simulink model "COSTEP_Auto"  (R2024b)
settings: Solver=FixedStepAuto  StartTime=0.0  StopTime=25  FixedStep=1/3600  RelTol=1e-3
model workspace (MAT data in the model file):
  AD : Simulink.Parameter (value not decoded)
  AG : Simulink.Parameter (value not decoded)
  AH : Simulink.Parameter (value not decoded)
  AV : Simulink.Parameter (value not decoded)
  AVP : Simulink.Parameter (value not decoded)
  BCHL : Simulink.Parameter (value not decoded)
  BCHV : Simulink.Parameter (value not decoded)
  BD : Simulink.Parameter (value not decoded)
  BG : Simulink.Parameter (value not decoded)
  BH : Simulink.Parameter (value not decoded)
  BVP : Simulink.Parameter (value not decoded)
  CD : Simulink.Parameter (value not decoded)
  CG : Simulink.Parameter (value not decoded)
  CH : Simulink.Parameter (value not decoded)
  CVP : Simulink.Parameter (value not decoded)
  ISV : Simulink.Parameter (value not decoded)
  XMW : Simulink.Parameter (value not decoded)
  XNS : Simulink.Parameter (value not decoded)
  XNS2 : Simulink.Parameter (value not decoded)
  XNS3 : Simulink.Parameter (value not decoded)
  XNSE : Simulink.Parameter (value not decoded)
values from neighbouring files (symbols this model uses):
  DD = SimData{4,1}{1,2}    [Auto_run_COSTEP.m]    (also in Run_COSTEP.m)
  G = SimData{2,1}(j,2)    [Auto_run_COSTEP.m]    (also in G.mat = [4243534565 7854912354 3456432354 1731738903 4346024432 5784; Run_COSTEP.m)
  IDV = SimData{3,1}(1:20,j)    [Auto_run_COSTEP.m]    (also in IDV.mat = [0 0 0 0 0 0 0 0 0 0 0 0 ... (812 elements, 28x29)]; Run_COSTEP.m = SimData{3,1}(1:28,j))
symbols that are objects in the model workspace (value not decoded): AD, AG, AH, AV, AVP, BD, BG, BH, BVP, CD, CG, CH, CVP, XMW, XNS, XNS2, XNS3, XNSE
undefined symbols (not defined in the file or in its folder): magnitude, msgbox, SETPT, XMEAS, XMV
libraries: mylib x304, dspindex x31
(part 11 of 13)

== system COSTEP_Auto/Control Mode/Ricker/Subsystem8/Control Loop 11/PI Control Measurement Velocity form/Subsystem ==
  Setpoint : Inport
  Measurement : Inport  Port=2
  Controller Gain : Gain  Gain=Kc  SaturateOnIntegerOverflow=on  OutDataTypeStr=Inherit: Same as input  ParamDataTypeStr=Inherit: Same as input
  Error : ZeroOrderHold  SampleTime=Ts
  Error old : UnitDelay  SampleTime=Ts
  Gain1 : Gain  Gain=Ts/Ti  SaturateOnIntegerOverflow=on  OutDataTypeStr=Inherit: Same as input  ParamDataTypeStr=Inherit: Same as input
  Sum : Sum  Inputs=|+-  SaturateOnIntegerOverflow=on
  Sum1 : Sum  Inputs=++-  SaturateOnIntegerOverflow=on
  Delta Output : Outport
  wires:
  Measurement/1 -> Sum/2
  Controller Gain/1 -> Delta Output/1
  Gain1/1 -> Sum1/2
  Setpoint/1 -> Sum/1
  Error old/1 -> Sum1/3
  Sum1/1 -> Controller Gain/1
  Error/1 -> Sum1/1, Error old/1, Gain1/1
  Sum/1 -> Error/1

== system COSTEP_Auto/Random number generator/Stream Measurements SMEAS Gas analysis/If Action Subsystem3/Subsystem/Stream 1/Subsystem ==
  G : Inport
  TESUB6 XMNSEA : Subsystem
  TESUB6 XMNSEB : Subsystem
  TESUB6 XMNSEC : Subsystem
  TESUB6 XMNSED : Subsystem
  TESUB6 XMNSEE : Subsystem
  TESUB6 XMNSEF : Subsystem
  TESUB6 XMNSEG : Subsystem
  TESUB6 XMNSEH : Subsystem
  XMNSEA : Outport  VectorParamsAs1DForOutWhenUnconnected=off
  XMNSEB : Outport  Port=2  VectorParamsAs1DForOutWhenUnconnected=off
  XMNSEC : Outport  Port=3  VectorParamsAs1DForOutWhenUnconnected=off
  XMNSED : Outport  Port=4  VectorParamsAs1DForOutWhenUnconnected=off
  XMNSEE : Outport  Port=5  VectorParamsAs1DForOutWhenUnconnected=off
  XMNSEF : Outport  Port=6  VectorParamsAs1DForOutWhenUnconnected=off
  XMNSEG : Outport  Port=7  VectorParamsAs1DForOutWhenUnconnected=off
  XMNSEH : Outport  Port=8  VectorParamsAs1DForOutWhenUnconnected=off
  G_NEW : Outport  Port=9  VectorParamsAs1DForOutWhenUnconnected=off
  wires:
  TESUB6 XMNSEB/2(G_NEW) -> TESUB6 XMNSEC/1(G)
  G/1 -> TESUB6 XMNSEA/1(G)
  TESUB6 XMNSEA/2(G_NEW) -> TESUB6 XMNSEB/1(G)
  TESUB6 XMNSEC/2(G_NEW) -> TESUB6 XMNSED/1(G)
  TESUB6 XMNSED/1(XMNSED) -> XMNSED/1  "XMNSED"
  TESUB6 XMNSEE/1(XMNSEE) -> XMNSEE/1  "XMNSEE"
  TESUB6 XMNSED/2(G_NEW) -> TESUB6 XMNSEE/1(G)
  TESUB6 XMNSEC/1(XMNSEC) -> XMNSEC/1  "XMNSEC"
  TESUB6 XMNSEA/1(XMNSEA) -> XMNSEA/1  "XMNSEA"
  TESUB6 XMNSEB/1(XMNSEB) -> XMNSEB/1  "XMNSEB"
  TESUB6 XMNSEE/2(G_NEW) -> TESUB6 XMNSEF/1(G)
  TESUB6 XMNSEF/2(G_NEW) -> TESUB6 XMNSEG/1(G)
  TESUB6 XMNSEG/2(G_NEW) -> TESUB6 XMNSEH/1(G)
  TESUB6 XMNSEH/2(G_NEW) -> G_NEW/1
  TESUB6 XMNSEF/1(XMNSEF) -> XMNSEF/1  "XMNSEF"
  TESUB6 XMNSEG/1(XMNSEG) -> XMNSEG/1  "XMNSEG"
  TESUB6 XMNSEH/1(XMNSEH) -> XMNSEH/1  "XMNSEH"

== system COSTEP_Auto/Random number generator/Stream Measurements SMEAS Gas analysis/If Action Subsystem3/Subsystem/Stream 13/Subsystem ==
  G : Inport
  TESUB6 XMNSEA : Subsystem
  TESUB6 XMNSEB : Subsystem
  TESUB6 XMNSEC : Subsystem
  TESUB6 XMNSED : Subsystem
  TESUB6 XMNSEE : Subsystem
  TESUB6 XMNSEF : Subsystem
  TESUB6 XMNSEG : Subsystem
  TESUB6 XMNSEH : Subsystem
  XMNSEA : Outport  VectorParamsAs1DForOutWhenUnconnected=off
  XMNSEB : Outport  Port=2  VectorParamsAs1DForOutWhenUnconnected=off
  XMNSEC : Outport  Port=3  VectorParamsAs1DForOutWhenUnconnected=off
  XMNSED : Outport  Port=4  VectorParamsAs1DForOutWhenUnconnected=off
  XMNSEE : Outport  Port=5  VectorParamsAs1DForOutWhenUnconnected=off
  XMNSEF : Outport  Port=6  VectorParamsAs1DForOutWhenUnconnected=off
  XMNSEG : Outport  Port=7  VectorParamsAs1DForOutWhenUnconnected=off
  XMNSEH : Outport  Port=8  VectorParamsAs1DForOutWhenUnconnected=off
  G_NEW : Outport  Port=9  VectorParamsAs1DForOutWhenUnconnected=off
  wires:
  TESUB6 XMNSEB/2(G_NEW) -> TESUB6 XMNSEC/1(G)
  G/1 -> TESUB6 XMNSEA/1(G)
  TESUB6 XMNSEA/2(G_NEW) -> TESUB6 XMNSEB/1(G)
  TESUB6 XMNSEC/2(G_NEW) -> TESUB6 XMNSED/1(G)
  TESUB6 XMNSED/1(XMNSED) -> XMNSED/1  "XMNSED"
  TESUB6 XMNSEE/1(XMNSEE) -> XMNSEE/1  "XMNSEE"
  TESUB6 XMNSED/2(G_NEW) -> TESUB6 XMNSEE/1(G)
  TESUB6 XMNSEC/1(XMNSEC) -> XMNSEC/1  "XMNSEC"
  TESUB6 XMNSEA/1(XMNSEA) -> XMNSEA/1  "XMNSEA"
  TESUB6 XMNSEB/1(XMNSEB) -> XMNSEB/1  "XMNSEB"
  TESUB6 XMNSEE/2(G_NEW) -> TESUB6 XMNSEF/1(G)
  TESUB6 XMNSEF/2(G_NEW) -> TESUB6 XMNSEG/1(G)
  TESUB6 XMNSEG/2(G_NEW) -> TESUB6 XMNSEH/1(G)
  TESUB6 XMNSEH/2(G_NEW) -> G_NEW/1
  TESUB6 XMNSEF/1(XMNSEF) -> XMNSEF/1  "XMNSEF"
  TESUB6 XMNSEG/1(XMNSEG) -> XMNSEG/1  "XMNSEG"
  TESUB6 XMNSEH/1(XMNSEH) -> XMNSEH/1  "XMNSEH"

== system COSTEP_Auto/Random number generator/Stream Measurements SMEAS Gas analysis/If Action Subsystem3/Subsystem/Stream 2/Subsystem ==
  G : Inport
  TESUB6 XMNSEA : Subsystem
  TESUB6 XMNSEB : Subsystem
  TESUB6 XMNSEC : Subsystem
  TESUB6 XMNSED : Subsystem
  TESUB6 XMNSEE : Subsystem
  TESUB6 XMNSEF : Subsystem
  TESUB6 XMNSEG : Subsystem
  TESUB6 XMNSEH : Subsystem
  XMNSEA : Outport  VectorParamsAs1DForOutWhenUnconnected=off
  XMNSEB : Outport  Port=2  VectorParamsAs1DForOutWhenUnconnected=off
  XMNSEC : Outport  Port=3  VectorParamsAs1DForOutWhenUnconnected=off
  XMNSED : Outport  Port=4  VectorParamsAs1DForOutWhenUnconnected=off
  XMNSEE : Outport  Port=5  VectorParamsAs1DForOutWhenUnconnected=off
  XMNSEF : Outport  Port=6  VectorParamsAs1DForOutWhenUnconnected=off
  XMNSEG : Outport  Port=7  VectorParamsAs1DForOutWhenUnconnected=off
  XMNSEH : Outport  Port=8  VectorParamsAs1DForOutWhenUnconnected=off
  G_NEW : Outport  Port=9  VectorParamsAs1DForOutWhenUnconnected=off
  wires:
  TESUB6 XMNSEB/2(G_NEW) -> TESUB6 XMNSEC/1(G)
  G/1 -> TESUB6 XMNSEA/1(G)
  TESUB6 XMNSEA/2(G_NEW) -> TESUB6 XMNSEB/1(G)
  TESUB6 XMNSEC/2(G_NEW) -> TESUB6 XMNSED/1(G)
  TESUB6 XMNSED/1(XMNSED) -> XMNSED/1  "XMNSED"
  TESUB6 XMNSEE/1(XMNSEE) -> XMNSEE/1  "XMNSEE"
  TESUB6 XMNSED/2(G_NEW) -> TESUB6 XMNSEE/1(G)
  TESUB6 XMNSEC/1(XMNSEC) -> XMNSEC/1  "XMNSEC"
  TESUB6 XMNSEA/1(XMNSEA) -> XMNSEA/1  "XMNSEA"
  TESUB6 XMNSEB/1(XMNSEB) -> XMNSEB/1  "XMNSEB"
  TESUB6 XMNSEE/2(G_NEW) -> TESUB6 XMNSEF/1(G)
  TESUB6 XMNSEF/2(G_NEW) -> TESUB6 XMNSEG/1(G)
  TESUB6 XMNSEG/2(G_NEW) -> TESUB6 XMNSEH/1(G)
  TESUB6 XMNSEH/2(G_NEW) -> G_NEW/1
  TESUB6 XMNSEF/1(XMNSEF) -> XMNSEF/1  "XMNSEF"
  TESUB6 XMNSEG/1(XMNSEG) -> XMNSEG/1  "XMNSEG"
  TESUB6 XMNSEH/1(XMNSEH) -> XMNSEH/1  "XMNSEH"

== system COSTEP_Auto/Random number generator/Stream Measurements SMEAS Gas analysis/If Action Subsystem3/Subsystem/Stream 3/Subsystem ==
  G : Inport
  TESUB6 XMNSEA : Subsystem
  TESUB6 XMNSEB : Subsystem
  TESUB6 XMNSEC : Subsystem
  TESUB6 XMNSED : Subsystem
  TESUB6 XMNSEE : Subsystem
  TESUB6 XMNSEF : Subsystem
  TESUB6 XMNSEG : Subsystem
  TESUB6 XMNSEH : Subsystem
  XMNSEA : Outport  VectorParamsAs1DForOutWhenUnconnected=off
  XMNSEB : Outport  Port=2  VectorParamsAs1DForOutWhenUnconnected=off
  XMNSEC : Outport  Port=3  VectorParamsAs1DForOutWhenUnconnected=off
  XMNSED : Outport  Port=4  VectorParamsAs1DForOutWhenUnconnected=off
  XMNSEE : Outport  Port=5  VectorParamsAs1DForOutWhenUnconnected=off
  XMNSEF : Outport  Port=6  VectorParamsAs1DForOutWhenUnconnected=off
  XMNSEG : Outport  Port=7  VectorParamsAs1DForOutWhenUnconnected=off
  XMNSEH : Outport  Port=8  VectorParamsAs1DForOutWhenUnconnected=off
  G_NEW : Outport  Port=9  VectorParamsAs1DForOutWhenUnconnected=off
  wires:
  TESUB6 XMNSEB/2(G_NEW) -> TESUB6 XMNSEC/1(G)
  G/1 -> TESUB6 XMNSEA/1(G)
  TESUB6 XMNSEA/2(G_NEW) -> TESUB6 XMNSEB/1(G)
  TESUB6 XMNSEC/2(G_NEW) -> TESUB6 XMNSED/1(G)
  TESUB6 XMNSED/1(XMNSED) -> XMNSED/1  "XMNSED"
  TESUB6 XMNSEE/1(XMNSEE) -> XMNSEE/1  "XMNSEE"
  TESUB6 XMNSED/2(G_NEW) -> TESUB6 XMNSEE/1(G)
  TESUB6 XMNSEC/1(XMNSEC) -> XMNSEC/1  "XMNSEC"
  TESUB6 XMNSEA/1(XMNSEA) -> XMNSEA/1  "XMNSEA"
  TESUB6 XMNSEB/1(XMNSEB) -> XMNSEB/1  "XMNSEB"
  TESUB6 XMNSEE/2(G_NEW) -> TESUB6 XMNSEF/1(G)
  TESUB6 XMNSEF/2(G_NEW) -> TESUB6 XMNSEG/1(G)
  TESUB6 XMNSEG/2(G_NEW) -> TESUB6 XMNSEH/1(G)
  TESUB6 XMNSEH/2(G_NEW) -> G_NEW/1
  TESUB6 XMNSEF/1(XMNSEF) -> XMNSEF/1  "XMNSEF"
  TESUB6 XMNSEG/1(XMNSEG) -> XMNSEG/1  "XMNSEG"
  TESUB6 XMNSEH/1(XMNSEH) -> XMNSEH/1  "XMNSEH"

== system COSTEP_Auto/Random number generator/Stream Measurements SMEAS Gas analysis/If Action Subsystem3/Subsystem/Stream 4/Subsystem ==
  G : Inport
  TESUB6 XMNSEA : Subsystem
  TESUB6 XMNSEB : Subsystem
  TESUB6 XMNSEC : Subsystem
  TESUB6 XMNSED : Subsystem
  TESUB6 XMNSEE : Subsystem
  TESUB6 XMNSEF : Subsystem
  TESUB6 XMNSEG : Subsystem
  TESUB6 XMNSEH : Subsystem
  XMNSEA : Outport  VectorParamsAs1DForOutWhenUnconnected=off
  XMNSEB : Outport  Port=2  VectorParamsAs1DForOutWhenUnconnected=off
  XMNSEC : Outport  Port=3  VectorParamsAs1DForOutWhenUnconnected=off
  XMNSED : Outport  Port=4  VectorParamsAs1DForOutWhenUnconnected=off
  XMNSEE : Outport  Port=5  VectorParamsAs1DForOutWhenUnconnected=off
  XMNSEF : Outport  Port=6  VectorParamsAs1DForOutWhenUnconnected=off
  XMNSEG : Outport  Port=7  VectorParamsAs1DForOutWhenUnconnected=off
  XMNSEH : Outport  Port=8  VectorParamsAs1DForOutWhenUnconnected=off
  G_NEW : Outport  Port=9  VectorParamsAs1DForOutWhenUnconnected=off
  wires:
  TESUB6 XMNSEB/2(G_NEW) -> TESUB6 XMNSEC/1(G)
  G/1 -> TESUB6 XMNSEA/1(G)
  TESUB6 XMNSEA/2(G_NEW) -> TESUB6 XMNSEB/1(G)
  TESUB6 XMNSEC/2(G_NEW) -> TESUB6 XMNSED/1(G)
  TESUB6 XMNSED/1(XMNSED) -> XMNSED/1  "XMNSED"
  TESUB6 XMNSEE/1(XMNSEE) -> XMNSEE/1  "XMNSEE"
  TESUB6 XMNSED/2(G_NEW) -> TESUB6 XMNSEE/1(G)
  TESUB6 XMNSEC/1(XMNSEC) -> XMNSEC/1  "XMNSEC"
  TESUB6 XMNSEA/1(XMNSEA) -> XMNSEA/1  "XMNSEA"
  TESUB6 XMNSEB/1(XMNSEB) -> XMNSEB/1  "XMNSEB"
  TESUB6 XMNSEE/2(G_NEW) -> TESUB6 XMNSEF/1(G)
  TESUB6 XMNSEF/2(G_NEW) -> TESUB6 XMNSEG/1(G)
  TESUB6 XMNSEG/2(G_NEW) -> TESUB6 XMNSEH/1(G)
  TESUB6 XMNSEH/2(G_NEW) -> G_NEW/1
  TESUB6 XMNSEF/1(XMNSEF) -> XMNSEF/1  "XMNSEF"
  TESUB6 XMNSEG/1(XMNSEG) -> XMNSEG/1  "XMNSEG"
  TESUB6 XMNSEH/1(XMNSEH) -> XMNSEH/1  "XMNSEH"

== system COSTEP_Auto/Random number generator/Stream Measurements SMEAS Gas analysis/If Action Subsystem3/Subsystem/Stream 5/Subsystem ==
  G : Inport
  TESUB6 XMNSEA : Subsystem
  TESUB6 XMNSEB : Subsystem
  TESUB6 XMNSEC : Subsystem
  TESUB6 XMNSED : Subsystem
  TESUB6 XMNSEE : Subsystem
  TESUB6 XMNSEF : Subsystem
  TESUB6 XMNSEG : Subsystem
  TESUB6 XMNSEH : Subsystem
  XMNSEA : Outport  VectorParamsAs1DForOutWhenUnconnected=off
  XMNSEB : Outport  Port=2  VectorParamsAs1DForOutWhenUnconnected=off
  XMNSEC : Outport  Port=3  VectorParamsAs1DForOutWhenUnconnected=off
  XMNSED : Outport  Port=4  VectorParamsAs1DForOutWhenUnconnected=off
  XMNSEE : Outport  Port=5  VectorParamsAs1DForOutWhenUnconnected=off
  XMNSEF : Outport  Port=6  VectorParamsAs1DForOutWhenUnconnected=off
  XMNSEG : Outport  Port=7  VectorParamsAs1DForOutWhenUnconnected=off
  XMNSEH : Outport  Port=8  VectorParamsAs1DForOutWhenUnconnected=off
  G_NEW : Outport  Port=9  VectorParamsAs1DForOutWhenUnconnected=off
  wires:
  TESUB6 XMNSEB/2(G_NEW) -> TESUB6 XMNSEC/1(G)
  G/1 -> TESUB6 XMNSEA/1(G)
  TESUB6 XMNSEA/2(G_NEW) -> TESUB6 XMNSEB/1(G)
  TESUB6 XMNSEC/2(G_NEW) -> TESUB6 XMNSED/1(G)
  TESUB6 XMNSED/1(XMNSED) -> XMNSED/1  "XMNSED"
  TESUB6 XMNSEE/1(XMNSEE) -> XMNSEE/1  "XMNSEE"
  TESUB6 XMNSED/2(G_NEW) -> TESUB6 XMNSEE/1(G)
  TESUB6 XMNSEC/1(XMNSEC) -> XMNSEC/1  "XMNSEC"
  TESUB6 XMNSEA/1(XMNSEA) -> XMNSEA/1  "XMNSEA"
  TESUB6 XMNSEB/1(XMNSEB) -> XMNSEB/1  "XMNSEB"
  TESUB6 XMNSEE/2(G_NEW) -> TESUB6 XMNSEF/1(G)
  TESUB6 XMNSEF/2(G_NEW) -> TESUB6 XMNSEG/1(G)
  TESUB6 XMNSEG/2(G_NEW) -> TESUB6 XMNSEH/1(G)
  TESUB6 XMNSEH/2(G_NEW) -> G_NEW/1
  TESUB6 XMNSEF/1(XMNSEF) -> XMNSEF/1  "XMNSEF"
  TESUB6 XMNSEG/1(XMNSEG) -> XMNSEG/1  "XMNSEG"
  TESUB6 XMNSEH/1(XMNSEH) -> XMNSEH/1  "XMNSEH"

== system COSTEP_Auto/Random number generator/Stream Measurements SMEAS Gas analysis/If Action Subsystem3/Subsystem/Stream 6/Subsystem ==
  G : Inport
  TESUB6 XMNSEA : Subsystem
  TESUB6 XMNSEB : Subsystem
  TESUB6 XMNSEC : Subsystem
  TESUB6 XMNSED : Subsystem
  TESUB6 XMNSEE : Subsystem
  TESUB6 XMNSEF : Subsystem
  TESUB6 XMNSEG : Subsystem
  TESUB6 XMNSEH : Subsystem
  XMNSEA : Outport  VectorParamsAs1DForOutWhenUnconnected=off
  XMNSEB : Outport  Port=2  VectorParamsAs1DForOutWhenUnconnected=off
  XMNSEC : Outport  Port=3  VectorParamsAs1DForOutWhenUnconnected=off
  XMNSED : Outport  Port=4  VectorParamsAs1DForOutWhenUnconnected=off
  XMNSEE : Outport  Port=5  VectorParamsAs1DForOutWhenUnconnected=off
  XMNSEF : Outport  Port=6  VectorParamsAs1DForOutWhenUnconnected=off
  XMNSEG : Outport  Port=7  VectorParamsAs1DForOutWhenUnconnected=off
  XMNSEH : Outport  Port=8  VectorParamsAs1DForOutWhenUnconnected=off
  G_NEW : Outport  Port=9  VectorParamsAs1DForOutWhenUnconnected=off
  wires:
  TESUB6 XMNSEB/2(G_NEW) -> TESUB6 XMNSEC/1(G)
  G/1 -> TESUB6 XMNSEA/1(G)
  TESUB6 XMNSEA/2(G_NEW) -> TESUB6 XMNSEB/1(G)
  TESUB6 XMNSEC/2(G_NEW) -> TESUB6 XMNSED/1(G)
  TESUB6 XMNSED/1(XMNSED) -> XMNSED/1  "XMNSED"
  TESUB6 XMNSEE/1(XMNSEE) -> XMNSEE/1  "XMNSEE"
  TESUB6 XMNSED/2(G_NEW) -> TESUB6 XMNSEE/1(G)
  TESUB6 XMNSEC/1(XMNSEC) -> XMNSEC/1  "XMNSEC"
  TESUB6 XMNSEA/1(XMNSEA) -> XMNSEA/1  "XMNSEA"
  TESUB6 XMNSEB/1(XMNSEB) -> XMNSEB/1  "XMNSEB"
  TESUB6 XMNSEE/2(G_NEW) -> TESUB6 XMNSEF/1(G)
  TESUB6 XMNSEF/2(G_NEW) -> TESUB6 XMNSEG/1(G)
  TESUB6 XMNSEG/2(G_NEW) -> TESUB6 XMNSEH/1(G)
  TESUB6 XMNSEH/2(G_NEW) -> G_NEW/1
  TESUB6 XMNSEF/1(XMNSEF) -> XMNSEF/1  "XMNSEF"
  TESUB6 XMNSEG/1(XMNSEG) -> XMNSEG/1  "XMNSEG"
  TESUB6 XMNSEH/1(XMNSEH) -> XMNSEH/1  "XMNSEH"

== system COSTEP_Auto/Random number generator/Stream Measurements SMEAS Gas analysis/If Action Subsystem3/Subsystem/Stream 8/Subsystem ==
  G : Inport
  TESUB6 XMNSEA : Subsystem
  TESUB6 XMNSEB : Subsystem
  TESUB6 XMNSEC : Subsystem
  TESUB6 XMNSED : Subsystem
  TESUB6 XMNSEE : Subsystem
  TESUB6 XMNSEF : Subsystem
  TESUB6 XMNSEG : Subsystem
  TESUB6 XMNSEH : Subsystem
  XMNSEA : Outport  VectorParamsAs1DForOutWhenUnconnected=off
  XMNSEB : Outport  Port=2  VectorParamsAs1DForOutWhenUnconnected=off
  XMNSEC : Outport  Port=3  VectorParamsAs1DForOutWhenUnconnected=off
  XMNSED : Outport  Port=4  VectorParamsAs1DForOutWhenUnconnected=off
  XMNSEE : Outport  Port=5  VectorParamsAs1DForOutWhenUnconnected=off
  XMNSEF : Outport  Port=6  VectorParamsAs1DForOutWhenUnconnected=off
  XMNSEG : Outport  Port=7  VectorParamsAs1DForOutWhenUnconnected=off
  XMNSEH : Outport  Port=8  VectorParamsAs1DForOutWhenUnconnected=off
  G_NEW : Outport  Port=9  VectorParamsAs1DForOutWhenUnconnected=off
  wires:
  TESUB6 XMNSEB/2(G_NEW) -> TESUB6 XMNSEC/1(G)
  G/1 -> TESUB6 XMNSEA/1(G)
  TESUB6 XMNSEA/2(G_NEW) -> TESUB6 XMNSEB/1(G)
  TESUB6 XMNSEC/2(G_NEW) -> TESUB6 XMNSED/1(G)
  TESUB6 XMNSED/1(XMNSED) -> XMNSED/1  "XMNSED"
  TESUB6 XMNSEE/1(XMNSEE) -> XMNSEE/1  "XMNSEE"
  TESUB6 XMNSED/2(G_NEW) -> TESUB6 XMNSEE/1(G)
  TESUB6 XMNSEC/1(XMNSEC) -> XMNSEC/1  "XMNSEC"
  TESUB6 XMNSEA/1(XMNSEA) -> XMNSEA/1  "XMNSEA"
  TESUB6 XMNSEB/1(XMNSEB) -> XMNSEB/1  "XMNSEB"
  TESUB6 XMNSEE/2(G_NEW) -> TESUB6 XMNSEF/1(G)
  TESUB6 XMNSEF/2(G_NEW) -> TESUB6 XMNSEG/1(G)
  TESUB6 XMNSEG/2(G_NEW) -> TESUB6 XMNSEH/1(G)
  TESUB6 XMNSEH/2(G_NEW) -> G_NEW/1
  TESUB6 XMNSEF/1(XMNSEF) -> XMNSEF/1  "XMNSEF"
  TESUB6 XMNSEG/1(XMNSEG) -> XMNSEG/1  "XMNSEG"
  TESUB6 XMNSEH/1(XMNSEH) -> XMNSEH/1  "XMNSEH"

== system COSTEP_Auto/Random number generator/Stream Measurements SMEAS Gas analysis/If Action Subsystem3/Subsystem/Stream 9/Subsystem ==
  G : Inport
  TESUB6 XMNSEA : Subsystem
  TESUB6 XMNSEB : Subsystem
  TESUB6 XMNSEC : Subsystem
  TESUB6 XMNSED : Subsystem
  TESUB6 XMNSEE : Subsystem
  TESUB6 XMNSEF : Subsystem
  TESUB6 XMNSEG : Subsystem
  TESUB6 XMNSEH : Subsystem
  XMNSEA : Outport  VectorParamsAs1DForOutWhenUnconnected=off
  XMNSEB : Outport  Port=2  VectorParamsAs1DForOutWhenUnconnected=off
  XMNSEC : Outport  Port=3  VectorParamsAs1DForOutWhenUnconnected=off
  XMNSED : Outport  Port=4  VectorParamsAs1DForOutWhenUnconnected=off
  XMNSEE : Outport  Port=5  VectorParamsAs1DForOutWhenUnconnected=off
  XMNSEF : Outport  Port=6  VectorParamsAs1DForOutWhenUnconnected=off
  XMNSEG : Outport  Port=7  VectorParamsAs1DForOutWhenUnconnected=off
  XMNSEH : Outport  Port=8  VectorParamsAs1DForOutWhenUnconnected=off
  G_NEW : Outport  Port=9  VectorParamsAs1DForOutWhenUnconnected=off
  wires:
  TESUB6 XMNSEB/2(G_NEW) -> TESUB6 XMNSEC/1(G)
  G/1 -> TESUB6 XMNSEA/1(G)
  TESUB6 XMNSEA/2(G_NEW) -> TESUB6 XMNSEB/1(G)
  TESUB6 XMNSEC/2(G_NEW) -> TESUB6 XMNSED/1(G)
  TESUB6 XMNSED/1(XMNSED) -> XMNSED/1  "XMNSED"
  TESUB6 XMNSEE/1(XMNSEE) -> XMNSEE/1  "XMNSEE"
  TESUB6 XMNSED/2(G_NEW) -> TESUB6 XMNSEE/1(G)
  TESUB6 XMNSEC/1(XMNSEC) -> XMNSEC/1  "XMNSEC"
  TESUB6 XMNSEA/1(XMNSEA) -> XMNSEA/1  "XMNSEA"
  TESUB6 XMNSEB/1(XMNSEB) -> XMNSEB/1  "XMNSEB"
  TESUB6 XMNSEE/2(G_NEW) -> TESUB6 XMNSEF/1(G)
  TESUB6 XMNSEF/2(G_NEW) -> TESUB6 XMNSEG/1(G)
  TESUB6 XMNSEG/2(G_NEW) -> TESUB6 XMNSEH/1(G)
  TESUB6 XMNSEH/2(G_NEW) -> G_NEW/1
  TESUB6 XMNSEF/1(XMNSEF) -> XMNSEF/1  "XMNSEF"
  TESUB6 XMNSEG/1(XMNSEG) -> XMNSEG/1  "XMNSEG"
  TESUB6 XMNSEH/1(XMNSEH) -> XMNSEH/1  "XMNSEH"

== system COSTEP_Auto/Random number generator/Stream Measurements SMEAS Product analysis/If Action Subsystem3/Subsystem/Subsystem1/Subsystem ==
  G : Inport
  TESUB6 XMNSED : Subsystem
  TESUB6 XMNSEE : Subsystem
  TESUB6 XMNSEF : Subsystem
  TESUB6 XMNSEG : Subsystem
  TESUB6 XMNSEH : Subsystem
  XMNSED : Outport  VectorParamsAs1DForOutWhenUnconnected=off
  XMNSEE : Outport  Port=2  VectorParamsAs1DForOutWhenUnconnected=off
  XMNSEF : Outport  Port=3  VectorParamsAs1DForOutWhenUnconnected=off
  XMNSEG : Outport  Port=4  VectorParamsAs1DForOutWhenUnconnected=off
  XMNSEH : Outport  Port=5  VectorParamsAs1DForOutWhenUnconnected=off
  G_NEW : Outport  Port=6  VectorParamsAs1DForOutWhenUnconnected=off
  wires:
  TESUB6 XMNSEE/2(G_NEW) -> TESUB6 XMNSEF/1(G)
  G/1 -> TESUB6 XMNSED/1(G)
  TESUB6 XMNSED/2(G_NEW) -> TESUB6 XMNSEE/1(G)
  TESUB6 XMNSEF/2(G_NEW) -> TESUB6 XMNSEG/1(G)
  TESUB6 XMNSEG/1(XMNS) -> XMNSEG/1  "XMNSEG"
  TESUB6 XMNSEH/1(XMNS) -> XMNSEH/1  "XMNSEH"
  TESUB6 XMNSEH/2(G_NEW) -> G_NEW/1
  TESUB6 XMNSEG/2(G_NEW) -> TESUB6 XMNSEH/1(G)
  TESUB6 XMNSEF/1(XMNS) -> XMNSEF/1  "XMNSEF"
  TESUB6 XMNSED/1(XMNS) -> XMNSED/1  "XMNSED"
  TESUB6 XMNSEE/1(XMNS) -> XMNSEE/1  "XMNSEE"

== system COSTEP_Auto/Random number generator/Stream Measurements SMEAS Product analysis/If Action Subsystem3/Subsystem/Subsystem2/Subsystem ==
  G : Inport
  TESUB6 XMNSED : Subsystem
  TESUB6 XMNSEE : Subsystem
  TESUB6 XMNSEF : Subsystem
  TESUB6 XMNSEG : Subsystem
  TESUB6 XMNSEH : Subsystem
  XMNSED : Outport  VectorParamsAs1DForOutWhenUnconnected=off
  XMNSEE : Outport  Port=2  VectorParamsAs1DForOutWhenUnconnected=off
  XMNSEF : Outport  Port=3  VectorParamsAs1DForOutWhenUnconnected=off
  XMNSEG : Outport  Port=4  VectorParamsAs1DForOutWhenUnconnected=off
  XMNSEH : Outport  Port=5  VectorParamsAs1DForOutWhenUnconnected=off
  G_NEW : Outport  Port=6  VectorParamsAs1DForOutWhenUnconnected=off
  wires:
  TESUB6 XMNSEE/2(G_NEW) -> TESUB6 XMNSEF/1(G)
  G/1 -> TESUB6 XMNSED/1(G)
  TESUB6 XMNSED/2(G_NEW) -> TESUB6 XMNSEE/1(G)
  TESUB6 XMNSEF/2(G_NEW) -> TESUB6 XMNSEG/1(G)
  TESUB6 XMNSEG/1(XMNS) -> XMNSEG/1  "XMNSEG"
  TESUB6 XMNSEH/1(XMNS) -> XMNSEH/1  "XMNSEH"
  TESUB6 XMNSEH/2(G_NEW) -> G_NEW/1
  TESUB6 XMNSEG/2(G_NEW) -> TESUB6 XMNSEH/1(G)
  TESUB6 XMNSEF/1(XMNS) -> XMNSEF/1  "XMNSEF"
  TESUB6 XMNSED/1(XMNS) -> XMNSED/1  "XMNSED"
  TESUB6 XMNSEE/1(XMNS) -> XMNSEE/1  "XMNSEE"

== system COSTEP_Auto/Stream Measurements/Subsystem6/A and C feed stream/Composition measurement mol%/Subsystem/Subsystem ==
  XST : Inport
  Constant : Constant  Value=100
  Multiport Selector : dspindex/Multiport Selector  rowsOrCols=Rows  idxCellArray={ 1,2,3}  idxErrMode=Clip Index
  Product : Product
  Product1 : Product
  Product2 : Product
  XCMPA : Outport  VectorParamsAs1DForOutWhenUnconnected=off
  XCMPB : Outport  Port=2  VectorParamsAs1DForOutWhenUnconnected=off
  XCMPC : Outport  Port=3  VectorParamsAs1DForOutWhenUnconnected=off
  wires:
  Multiport Selector/1 -> Product/1
  Multiport Selector/3 -> Product2/1
  Constant/1 -> Product/2, Product1/2, Product2/2
  XST/1 -> Multiport Selector/1
  Multiport Selector/2 -> Product1/1
  Product/1 -> XCMPA/1
  Product1/1 -> XCMPB/1
  Product2/1 -> XCMPC/1

== system COSTEP_Auto/Stream Measurements/Subsystem6/A feed stream/Composition measurement mol%/Subsystem/Subsystem ==
  XST : Inport
  Constant : Constant  Value=100
  Multiport Selector : dspindex/Multiport Selector  rowsOrCols=Rows  idxCellArray={ 1,2}  idxErrMode=Clip Index
  Product : Product
  Product1 : Product
  XCMPA : Outport  VectorParamsAs1DForOutWhenUnconnected=off
  XCMPB : Outport  Port=2  VectorParamsAs1DForOutWhenUnconnected=off
  wires:
  Multiport Selector/1 -> Product/1
  Constant/1 -> Product/2, Product1/2
  XST/1 -> Multiport Selector/1
  Multiport Selector/2 -> Product1/1
  Product/1 -> XCMPA/1
  Product1/1 -> XCMPB/1

== system COSTEP_Auto/Stream Measurements/Subsystem6/Condenser product stream/Composition measurement mol%/Subsystem/Subsystem ==
  XST : Inport
  Constant : Constant  Value=100
  Multiport Selector : dspindex/Multiport Selector  rowsOrCols=Rows  idxCellArray={ 1,2,3,4,5,6,7,8}  idxErrMode=Clip Index
  Product{,1..7} (8 alike) : Product
  XCMPA : Outport  VectorParamsAs1DForOutWhenUnconnected=off
  XCMPB : Outport  Port=2  VectorParamsAs1DForOutWhenUnconnected=off
  XCMPC : Outport  Port=3  VectorParamsAs1DForOutWhenUnconnected=off
  XCMPD : Outport  Port=4  VectorParamsAs1DForOutWhenUnconnected=off
  "XCMPE " : Outport  Port=5  VectorParamsAs1DForOutWhenUnconnected=off
  "XCMPF " : Outport  Port=6  VectorParamsAs1DForOutWhenUnconnected=off
  XCMPG : Outport  Port=7  VectorParamsAs1DForOutWhenUnconnected=off
  "XCMPH " : Outport  Port=8  VectorParamsAs1DForOutWhenUnconnected=off
  wires:
  Multiport Selector/6 -> Product5/1
  Multiport Selector/8 -> Product7/1
  Multiport Selector/5 -> Product4/1
  Multiport Selector/7 -> Product6/1
  Multiport Selector/1 -> Product/1
  Multiport Selector/3 -> Product2/1
  Constant/1 -> Product/2, Product1/2, Product2/2, Product3/2, Product4/2, Product5/2, Product7/2, Product6/2
  Multiport Selector/4 -> Product3/1
  XST/1 -> Multiport Selector/1
  Multiport Selector/2 -> Product1/1
  Product/1 -> XCMPA/1
  Product1/1 -> XCMPB/1
  Product2/1 -> XCMPC/1
  Product3/1 -> XCMPD/1
  Product4/1 -> "XCMPE "/1
  Product5/1 -> "XCMPF "/1
  Product6/1 -> XCMPG/1
  Product7/1 -> "XCMPH "/1

== system COSTEP_Auto/Stream Measurements/Subsystem6/D feed stream/Composition measurement mol%/Subsystem/Subsystem ==
  XST : Inport
  Constant : Constant  Value=100
  Multiport Selector : dspindex/Multiport Selector  rowsOrCols=Rows  idxCellArray={ 2,4}  idxErrMode=Clip Index
  Product : Product
  Product1 : Product
  XCMPB : Outport  VectorParamsAs1DForOutWhenUnconnected=off
  XCMPD : Outport  Port=2  VectorParamsAs1DForOutWhenUnconnected=off
  wires:
  Multiport Selector/1 -> Product/1
  Constant/1 -> Product/2, Product1/2
  XST/1 -> Multiport Selector/1
  Multiport Selector/2 -> Product1/1
  Product/1 -> XCMPB/1
  Product1/1 -> XCMPD/1

== system COSTEP_Auto/Stream Measurements/Subsystem6/E feed stream/Composition measurement mol%/Subsystem/Subsystem ==
  XST : Inport
  Constant : Constant  Value=100
  Multiport Selector : dspindex/Multiport Selector  rowsOrCols=Rows  idxCellArray={ 5,6}  idxErrMode=Clip Index
  Product : Product
  Product1 : Product
  "XCMPE " : Outport  VectorParamsAs1DForOutWhenUnconnected=off
  "XCMPF " : Outport  Port=2  VectorParamsAs1DForOutWhenUnconnected=off
  wires:
  Multiport Selector/1 -> Product/1
  Constant/1 -> Product/2, Product1/2
  XST/1 -> Multiport Selector/1
  Multiport Selector/2 -> Product1/1
  Product/1 -> "XCMPE "/1
  Product1/1 -> "XCMPF "/1

== system COSTEP_Auto/Stream Measurements/Subsystem6/Product stream/Composition measurement mol%/Subsystem/Subsystem ==
  XST : Inport
  Constant : Constant  Value=100
  Multiport Selector : dspindex/Multiport Selector  rowsOrCols=Rows  idxCellArray={ 1,2,3}  idxErrMode=Clip Index
  Product : Product
  Product1 : Product
  Product2 : Product
  XCMPA : Outport  VectorParamsAs1DForOutWhenUnconnected=off
  XCMPB : Outport  Port=2  VectorParamsAs1DForOutWhenUnconnected=off
  XCMPC : Outport  Port=3  VectorParamsAs1DForOutWhenUnconnected=off
  wires:
  Multiport Selector/1 -> Product/1
  Multiport Selector/3 -> Product2/1
  Constant/1 -> Product2/2, Product/2, Product1/2
  XST/1 -> Multiport Selector/1
  Multiport Selector/2 -> Product1/1
  Product/1 -> XCMPA/1
  Product1/1 -> XCMPB/1
  Product2/1 -> XCMPC/1

== system COSTEP_Auto/Stream Measurements/Subsystem6/Product stream/Composition measurement mol%/Subsystem1/Subsystem ==
  XST : Inport
  Constant : Constant  Value=100
  Multiport Selector : dspindex/Multiport Selector  rowsOrCols=Rows  idxCellArray={4,5,6,7,8}  idxErrMode=Clip Index
  "XCMPD " : Product
  XCMPE : Product
  XCMPF : Product
  "XCMPG " : Product
  XCMPH : Product
  XCMPD : Outport  VectorParamsAs1DForOutWhenUnconnected=off
  "XCMPE " : Outport  Port=2  VectorParamsAs1DForOutWhenUnconnected=off
  "XCMPF " : Outport  Port=3  VectorParamsAs1DForOutWhenUnconnected=off
  XCMPG : Outport  Port=4  VectorParamsAs1DForOutWhenUnconnected=off
  "XCMPH " : Outport  Port=5  VectorParamsAs1DForOutWhenUnconnected=off
  wires:
  Constant/1 -> XCMPE/2, "XCMPG "/2, XCMPH/2, XCMPF/2, "XCMPD "/2
  Multiport Selector/1 -> "XCMPD "/1
  "XCMPD "/1 -> XCMPD/1  "XCMPD"
  Multiport Selector/5 -> XCMPH/1
  XCMPF/1 -> "XCMPF "/1  "XCMPF"
  XST/1 -> Multiport Selector/1
  Multiport Selector/4 -> "XCMPG "/1
  Multiport Selector/2 -> XCMPE/1
  Multiport Selector/3 -> XCMPF/1
  XCMPE/1 -> "XCMPE "/1  "XCMPE"
  XCMPH/1 -> "XCMPH "/1  "XCMPH"
  "XCMPG "/1 -> XCMPG/1  "XCMPG"

== system COSTEP_Auto/Stream Measurements/Subsystem6/Reactor feed stream/Composition measurement mol%/Subsystem/Subsystem ==
  XST : Inport
  Constant : Constant  Value=100
  Multiport Selector : dspindex/Multiport Selector  rowsOrCols=Rows  idxCellArray={7,8}  idxErrMode=Clip Index
  Product6 : Product
  Product7 : Product
  XCMPG : Outport  VectorParamsAs1DForOutWhenUnconnected=off
  "XCMPH " : Outport  Port=2  VectorParamsAs1DForOutWhenUnconnected=off
  wires:
  Multiport Selector/2 -> Product7/1
  Multiport Selector/1 -> Product6/1
  Constant/1 -> Product6/2, Product7/2
  XST/1 -> Multiport Selector/1
  Product6/1 -> XCMPG/1
  Product7/1 -> "XCMPH "/1

== system COSTEP_Auto/Stream Measurements/Subsystem6/Reactor product stream/Composition measurement mol%/Subsystem/Subsystem ==
  XST : Inport
  Constant : Constant  Value=100
  Multiport Selector : dspindex/Multiport Selector  rowsOrCols=Rows  idxCellArray={ 1,2,3,4,5,6,7,8}  idxErrMode=Clip Index
  Product{,1..7} (8 alike) : Product
  XCMPA : Outport  VectorParamsAs1DForOutWhenUnconnected=off
  XCMPB : Outport  Port=2  VectorParamsAs1DForOutWhenUnconnected=off
  XCMPC : Outport  Port=3  VectorParamsAs1DForOutWhenUnconnected=off
  XCMPD : Outport  Port=4  VectorParamsAs1DForOutWhenUnconnected=off
  "XCMPE " : Outport  Port=5  VectorParamsAs1DForOutWhenUnconnected=off
  "XCMPF " : Outport  Port=6  VectorParamsAs1DForOutWhenUnconnected=off
  XCMPG : Outport  Port=7  VectorParamsAs1DForOutWhenUnconnected=off
  "XCMPH " : Outport  Port=8  VectorParamsAs1DForOutWhenUnconnected=off
  wires:
  Multiport Selector/6 -> Product5/1
  Multiport Selector/8 -> Product7/1
  Multiport Selector/5 -> Product4/1
  Multiport Selector/7 -> Product6/1
  Multiport Selector/1 -> Product/1
  Multiport Selector/3 -> Product2/1
  Constant/1 -> Product/2, Product1/2, Product2/2, Product3/2, Product4/2, Product5/2, Product7/2, Product6/2
  Multiport Selector/4 -> Product3/1
  XST/1 -> Multiport Selector/1
  Multiport Selector/2 -> Product1/1
  Product/1 -> XCMPA/1
  Product1/1 -> XCMPB/1
  Product2/1 -> XCMPC/1
  Product3/1 -> XCMPD/1
  Product4/1 -> "XCMPE "/1
  Product5/1 -> "XCMPF "/1
  Product6/1 -> XCMPG/1
  Product7/1 -> "XCMPH "/1

== system COSTEP_Auto/Stream Measurements/Subsystem6/Separator product stream/Composition measurement mol%/Subsystem/Subsystem ==
  XST : Inport
  Constant : Constant  Value=100
  Multiport Selector : dspindex/Multiport Selector  rowsOrCols=Rows  idxCellArray={ 1,2,3,4,5,6,7,8}  idxErrMode=Clip Index
  Product{,1..7} (8 alike) : Product
  XCMPA : Outport  VectorParamsAs1DForOutWhenUnconnected=off
  XCMPB : Outport  Port=2  VectorParamsAs1DForOutWhenUnconnected=off
  XCMPC : Outport  Port=3  VectorParamsAs1DForOutWhenUnconnected=off
  XCMPD : Outport  Port=4  VectorParamsAs1DForOutWhenUnconnected=off
  "XCMPE " : Outport  Port=5  VectorParamsAs1DForOutWhenUnconnected=off
  "XCMPF " : Outport  Port=6  VectorParamsAs1DForOutWhenUnconnected=off
  XCMPG : Outport  Port=7  VectorParamsAs1DForOutWhenUnconnected=off
  "XCMPH " : Outport  Port=8  VectorParamsAs1DForOutWhenUnconnected=off
  wires:
  Multiport Selector/6 -> Product5/1
  Multiport Selector/8 -> Product7/1
  Multiport Selector/5 -> Product4/1
  Multiport Selector/7 -> Product6/1
  Multiport Selector/1 -> Product/1
  Multiport Selector/3 -> Product2/1
  Constant/1 -> Product/2, Product1/2, Product2/2, Product3/2, Product4/2, Product5/2, Product7/2, Product6/2
  Multiport Selector/4 -> Product3/1
  XST/1 -> Multiport Selector/1
  Multiport Selector/2 -> Product1/1
  Product/1 -> XCMPA/1
  Product1/1 -> XCMPB/1
  Product2/1 -> XCMPC/1
  Product3/1 -> XCMPD/1
  Product4/1 -> "XCMPE "/1
  Product5/1 -> "XCMPF "/1
  Product6/1 -> XCMPG/1
  Product7/1 -> "XCMPH "/1

== system COSTEP_Auto/Stream Measurements/Subsystem6/Separator product stream/Flow measurement in kg//h/Subsystem/XMWS Molecular weight of Stream lb//lb-mol ==
  XST : Inport
  Product : Product
  Sum of Elements : Sum  Inputs=+
  "XMW(I) Molecular weight of components lb/lb-mol " : Constant  Value=XMW
  XMWS : Outport  VectorParamsAs1DForOutWhenUnconnected=off
  wires:
  Sum of Elements/1 -> XMWS/1
  Product/1 -> Sum of Elements/1
  XST/1 -> Product/1
  "XMW(I) Molecular weight of components lb/lb-mol "/1 -> Product/2

== system COSTEP_Auto/Stream Measurements/Subsystem6/Separator product stream/Flow measurement in kg//h/Subsystem1/XMWS Molecular weight of Stream lb//lb-mol ==
  XST : Inport
  Product : Product
  Sum of Elements : Sum  Inputs=+
  "XMW(I) Molecular weight of components lb/lb-mol " : Constant  Value=XMW
  XMWS : Outport  VectorParamsAs1DForOutWhenUnconnected=off
  wires:
  Sum of Elements/1 -> XMWS/1
  Product/1 -> Sum of Elements/1
  XST/1 -> Product/1
  "XMW(I) Molecular weight of components lb/lb-mol "/1 -> Product/2

== system COSTEP_Auto/Stream Measurements/Subsystem6/Separator recycle stream (after compressor)/Composition measurement mol%/Subsystem/Subsystem ==
  XST : Inport
  Constant : Constant  Value=100
  Multiport Selector : dspindex/Multiport Selector  rowsOrCols=Rows  idxCellArray={ 1,2,3,4,5,6,7,8}  idxErrMode=Clip Index
  Product{,1..7} (8 alike) : Product
  XCMPA : Outport  VectorParamsAs1DForOutWhenUnconnected=off
  XCMPB : Outport  Port=2  VectorParamsAs1DForOutWhenUnconnected=off
  XCMPC : Outport  Port=3  VectorParamsAs1DForOutWhenUnconnected=off
  XCMPD : Outport  Port=4  VectorParamsAs1DForOutWhenUnconnected=off
  "XCMPE " : Outport  Port=5  VectorParamsAs1DForOutWhenUnconnected=off
  "XCMPF " : Outport  Port=6  VectorParamsAs1DForOutWhenUnconnected=off
  XCMPG : Outport  Port=7  VectorParamsAs1DForOutWhenUnconnected=off
  "XCMPH " : Outport  Port=8  VectorParamsAs1DForOutWhenUnconnected=off
  wires:
  Multiport Selector/6 -> Product5/1
  Multiport Selector/8 -> Product7/1
  Multiport Selector/5 -> Product4/1
  Multiport Selector/7 -> Product6/1
  Multiport Selector/1 -> Product/1
  Multiport Selector/3 -> Product2/1
  Constant/1 -> Product/2, Product1/2, Product2/2, Product3/2, Product4/2, Product5/2, Product7/2, Product6/2
  Multiport Selector/4 -> Product3/1
  XST/1 -> Multiport Selector/1
  Multiport Selector/2 -> Product1/1
  Product/1 -> XCMPA/1
  Product1/1 -> XCMPB/1
  Product2/1 -> XCMPC/1
  Product3/1 -> XCMPD/1
  Product4/1 -> "XCMPE "/1
  Product5/1 -> "XCMPF "/1
  Product6/1 -> XCMPG/1
  Product7/1 -> "XCMPH "/1

== system COSTEP_Auto/Stream Measurements/Subsystem6/Separator recycle stream (before compressor)/Composition measurement mol%/Subsystem/Subsystem ==
  XST : Inport
  Constant : Constant  Value=100
  Multiport Selector : dspindex/Multiport Selector  rowsOrCols=Rows  idxCellArray={ 1,2,3,4,5,6,7,8}  idxErrMode=Clip Index
  Product{,1..7} (8 alike) : Product
  XCMPA : Outport  VectorParamsAs1DForOutWhenUnconnected=off
  XCMPB : Outport  Port=2  VectorParamsAs1DForOutWhenUnconnected=off
  XCMPC : Outport  Port=3  VectorParamsAs1DForOutWhenUnconnected=off
  XCMPD : Outport  Port=4  VectorParamsAs1DForOutWhenUnconnected=off
  "XCMPE " : Outport  Port=5  VectorParamsAs1DForOutWhenUnconnected=off
  "XCMPF " : Outport  Port=6  VectorParamsAs1DForOutWhenUnconnected=off
  XCMPG : Outport  Port=7  VectorParamsAs1DForOutWhenUnconnected=off
  "XCMPH " : Outport  Port=8  VectorParamsAs1DForOutWhenUnconnected=off
  wires:
  Multiport Selector/6 -> Product5/1
  Multiport Selector/8 -> Product7/1
  Multiport Selector/5 -> Product4/1
  Multiport Selector/7 -> Product6/1
  Multiport Selector/1 -> Product/1
  Multiport Selector/3 -> Product2/1
  Constant/1 -> Product/2, Product1/2, Product2/2, Product3/2, Product4/2, Product5/2, Product7/2, Product6/2
  Multiport Selector/4 -> Product3/1
  XST/1 -> Multiport Selector/1
  Multiport Selector/2 -> Product1/1
  Product/1 -> XCMPA/1
  Product1/1 -> XCMPB/1
  Product2/1 -> XCMPC/1
  Product3/1 -> XCMPD/1
  Product4/1 -> "XCMPE "/1
  Product5/1 -> "XCMPF "/1
  Product6/1 -> XCMPG/1
  Product7/1 -> "XCMPH "/1

== system COSTEP_Auto/Stream Measurements/Subsystem6/Separator underflow stream/Composition measurement mol%/Subsystem/Subsystem ==
  XST : Inport
  Constant : Constant  Value=100
  Multiport Selector : dspindex/Multiport Selector  rowsOrCols=Rows  idxCellArray={ 4,5,6,7,8}  idxErrMode=Clip Index
  Product{3..7} (5 alike) : Product
  XCMPD : Outport  VectorParamsAs1DForOutWhenUnconnected=off
  "XCMPE " : Outport  Port=2  VectorParamsAs1DForOutWhenUnconnected=off
  "XCMPF " : Outport  Port=3  VectorParamsAs1DForOutWhenUnconnected=off
  XCMPG : Outport  Port=4  VectorParamsAs1DForOutWhenUnconnected=off
  "XCMPH " : Outport  Port=5  VectorParamsAs1DForOutWhenUnconnected=off
  wires:
  Constant/1 -> Product3/2, Product4/2, Product5/2, Product7/2, Product6/2
  XST/1 -> Multiport Selector/1
  Product3/1 -> XCMPD/1
  Product4/1 -> "XCMPE "/1
  Product5/1 -> "XCMPF "/1
  Product6/1 -> XCMPG/1
  Product7/1 -> "XCMPH "/1
  Multiport Selector/1 -> Product3/1
  Multiport Selector/2 -> Product4/1
  Multiport Selector/3 -> Product5/1
  Multiport Selector/4 -> Product6/1
  Multiport Selector/5 -> Product7/1

== system COSTEP_Auto/Stream Measurements/Subsystem6/Stripper recycle stream/Composition measurement mol%/Subsystem/Subsystem ==
  XST : Inport
  Constant : Constant  Value=100
  Multiport Selector : dspindex/Multiport Selector  rowsOrCols=Rows  idxCellArray={ 1,2,3,4,5,6,7,8}  idxErrMode=Clip Index
  Product{,1..7} (8 alike) : Product
  XCMPA : Outport  VectorParamsAs1DForOutWhenUnconnected=off
  XCMPB : Outport  Port=2  VectorParamsAs1DForOutWhenUnconnected=off
  XCMPC : Outport  Port=3  VectorParamsAs1DForOutWhenUnconnected=off
  XCMPD : Outport  Port=4  VectorParamsAs1DForOutWhenUnconnected=off
  "XCMPE " : Outport  Port=5  VectorParamsAs1DForOutWhenUnconnected=off
  "XCMPF " : Outport  Port=6  VectorParamsAs1DForOutWhenUnconnected=off
  XCMPG : Outport  Port=7  VectorParamsAs1DForOutWhenUnconnected=off
  "XCMPH " : Outport  Port=8  VectorParamsAs1DForOutWhenUnconnected=off
  wires:
  Multiport Selector/6 -> Product5/1
  Multiport Selector/8 -> Product7/1
  Multiport Selector/5 -> Product4/1
  Multiport Selector/7 -> Product6/1
  Multiport Selector/1 -> Product/1
  Multiport Selector/3 -> Product2/1
  Constant/1 -> Product/2, Product1/2, Product2/2, Product3/2, Product4/2, Product5/2, Product7/2, Product6/2
  Multiport Selector/4 -> Product3/1
  XST/1 -> Multiport Selector/1
  Multiport Selector/2 -> Product1/1
  Product/1 -> XCMPA/1
  Product1/1 -> XCMPB/1
  Product2/1 -> XCMPC/1
  Product3/1 -> XCMPD/1
  Product4/1 -> "XCMPE "/1
  Product5/1 -> "XCMPF "/1
  Product6/1 -> XCMPG/1
  Product7/1 -> "XCMPH "/1

== system COSTEP_Auto/Control Mode/Braatz/ 10/CONTROL 6/P Control Velocity form/Pressure limits/If Action Subsystem ==
  In1 : Inport
  Action Port : ActionPort  ActionPortLabel=if(u1 >= 2950)
  Out1 : Outport  VectorParamsAs1DForOutWhenUnconnected=off
  wires:
  In1/1 -> Out1/1

== system COSTEP_Auto/Control Mode/Braatz/ 10/CONTROL 6/P Control Velocity form/Pressure limits/If Action Subsystem1 ==
  In1 : Inport
  Action Port : ActionPort  ActionPortLabel=elseif(u1 <= 2300)
  Out1 : Outport  VectorParamsAs1DForOutWhenUnconnected=off
  wires:
  In1/1 -> Out1/1

== system COSTEP_Auto/Control Mode/Braatz/ 10/CONTROL 6/P Control Velocity form/Pressure limits/If Action Subsystem2 ==
  In1 : Inport
  Action Port : ActionPort  ActionPortLabel=else
  Out1 : Outport  VectorParamsAs1DForOutWhenUnconnected=off
  wires:
  In1/1 -> Out1/1

== system COSTEP_Auto/Random number generator/Stream Measurements SMEAS Gas analysis/If Action Subsystem3/Subsystem/Stream 1/Subsystem/TESUB6 XMNSEA ==
  G : Inport
  Process Noise I=1-12 G New : mylib/Process Noise I=1-12 G New  SystemSampleTime=-1  VariantActivationTime=update diagram  AllowFlexibleInterface=on  Latency=0  AutoFrameSizeCalculation=off
  XNSEA : Constant  Value=0.25
  XMNSEA : Outport  VectorParamsAs1DForOutWhenUnconnected=off
  G_NEW : Outport  Port=2  VectorParamsAs1DForOutWhenUnconnected=off
  wires:
  XNSEA/1 -> Process Noise I=1-12 G New/1
  Process Noise I=1-12 G New/1 -> XMNSEA/1
  G/1 -> Process Noise I=1-12 G New/2
  Process Noise I=1-12 G New/2 -> G_NEW/1

== system COSTEP_Auto/Random number generator/Stream Measurements SMEAS Gas analysis/If Action Subsystem3/Subsystem/Stream 1/Subsystem/TESUB6 XMNSEB ==
  G : Inport
  Process Noise I=1-12 G New : mylib/Process Noise I=1-12 G New  SystemSampleTime=-1  VariantActivationTime=update diagram  AllowFlexibleInterface=on  Latency=0  AutoFrameSizeCalculation=off
  XNSEB : Constant  Value=0.1
  XMNSEB : Outport  VectorParamsAs1DForOutWhenUnconnected=off
  G_NEW : Outport  Port=2  VectorParamsAs1DForOutWhenUnconnected=off
  wires:
  XNSEB/1 -> Process Noise I=1-12 G New/1
  Process Noise I=1-12 G New/1 -> XMNSEB/1
  G/1 -> Process Noise I=1-12 G New/2
  Process Noise I=1-12 G New/2 -> G_NEW/1

== system COSTEP_Auto/Random number generator/Stream Measurements SMEAS Gas analysis/If Action Subsystem3/Subsystem/Stream 1/Subsystem/TESUB6 XMNSEC ==
  G : Inport
  Process Noise I=1-12 G New : mylib/Process Noise I=1-12 G New  SystemSampleTime=-1  VariantActivationTime=update diagram  AllowFlexibleInterface=on  Latency=0  AutoFrameSizeCalculation=off
  XNSEC : Constant  Value=0.25
  XMNSEC : Outport  VectorParamsAs1DForOutWhenUnconnected=off
  G_NEW : Outport  Port=2  VectorParamsAs1DForOutWhenUnconnected=off
  wires:
  XNSEC/1 -> Process Noise I=1-12 G New/1
  Process Noise I=1-12 G New/1 -> XMNSEC/1
  G/1 -> Process Noise I=1-12 G New/2
  Process Noise I=1-12 G New/2 -> G_NEW/1

== system COSTEP_Auto/Random number generator/Stream Measurements SMEAS Gas analysis/If Action Subsystem3/Subsystem/Stream 1/Subsystem/TESUB6 XMNSED ==
  G : Inport
  Process Noise I=1-12 G New : mylib/Process Noise I=1-12 G New  SystemSampleTime=-1  VariantActivationTime=update diagram  AllowFlexibleInterface=on  Latency=0  AutoFrameSizeCalculation=off
  XNSED : Constant  Value=0.1
  XMNSED : Outport  VectorParamsAs1DForOutWhenUnconnected=off
  G_NEW : Outport  Port=2  VectorParamsAs1DForOutWhenUnconnected=off
  wires:
  XNSED/1 -> Process Noise I=1-12 G New/1
  Process Noise I=1-12 G New/1 -> XMNSED/1
  G/1 -> Process Noise I=1-12 G New/2
  Process Noise I=1-12 G New/2 -> G_NEW/1

== system COSTEP_Auto/Random number generator/Stream Measurements SMEAS Gas analysis/If Action Subsystem3/Subsystem/Stream 1/Subsystem/TESUB6 XMNSEE ==
  G : Inport
  Process Noise I=1-12 G New : mylib/Process Noise I=1-12 G New  SystemSampleTime=-1  VariantActivationTime=update diagram  AllowFlexibleInterface=on  Latency=0  AutoFrameSizeCalculation=off
  XNSEE : Constant  Value=0.25
  XMNSEE : Outport  VectorParamsAs1DForOutWhenUnconnected=off
  G_NEW : Outport  Port=2  VectorParamsAs1DForOutWhenUnconnected=off
  wires:
  XNSEE/1 -> Process Noise I=1-12 G New/1
  Process Noise I=1-12 G New/1 -> XMNSEE/1
  G/1 -> Process Noise I=1-12 G New/2
  Process Noise I=1-12 G New/2 -> G_NEW/1

== system COSTEP_Auto/Random number generator/Stream Measurements SMEAS Gas analysis/If Action Subsystem3/Subsystem/Stream 1/Subsystem/TESUB6 XMNSEF ==
  G : Inport
  Process Noise I=1-12 G New : mylib/Process Noise I=1-12 G New  SystemSampleTime=-1  VariantActivationTime=update diagram  AllowFlexibleInterface=on  Latency=0  AutoFrameSizeCalculation=off
  XNSEF : Constant  Value=0.025
  XMNSEF : Outport  VectorParamsAs1DForOutWhenUnconnected=off
  G_NEW : Outport  Port=2  VectorParamsAs1DForOutWhenUnconnected=off
  wires:
  XNSEF/1 -> Process Noise I=1-12 G New/1
  Process Noise I=1-12 G New/1 -> XMNSEF/1
  G/1 -> Process Noise I=1-12 G New/2
  Process Noise I=1-12 G New/2 -> G_NEW/1

== system COSTEP_Auto/Random number generator/Stream Measurements SMEAS Gas analysis/If Action Subsystem3/Subsystem/Stream 1/Subsystem/TESUB6 XMNSEG ==
  G : Inport
  Process Noise I=1-12 G New : mylib/Process Noise I=1-12 G New  SystemSampleTime=-1  VariantActivationTime=update diagram  AllowFlexibleInterface=on  Latency=0  AutoFrameSizeCalculation=off
  XNSEG : Constant  Value=0.05
  XMNSEG : Outport  VectorParamsAs1DForOutWhenUnconnected=off
  G_NEW : Outport  Port=2  VectorParamsAs1DForOutWhenUnconnected=off
  wires:
  XNSEG/1 -> Process Noise I=1-12 G New/1
  Process Noise I=1-12 G New/1 -> XMNSEG/1
  G/1 -> Process Noise I=1-12 G New/2
  Process Noise I=1-12 G New/2 -> G_NEW/1

== system COSTEP_Auto/Random number generator/Stream Measurements SMEAS Gas analysis/If Action Subsystem3/Subsystem/Stream 1/Subsystem/TESUB6 XMNSEH ==
  G : Inport
  Process Noise I=1-12 G New : mylib/Process Noise I=1-12 G New  SystemSampleTime=-1  VariantActivationTime=update diagram  AllowFlexibleInterface=on  Latency=0  AutoFrameSizeCalculation=off
  XNSEH : Constant  Value=0.05
  XMNSEH : Outport  VectorParamsAs1DForOutWhenUnconnected=off
  G_NEW : Outport  Port=2  VectorParamsAs1DForOutWhenUnconnected=off
  wires:
  XNSEH/1 -> Process Noise I=1-12 G New/1
  Process Noise I=1-12 G New/1 -> XMNSEH/1
  G/1 -> Process Noise I=1-12 G New/2
  Process Noise I=1-12 G New/2 -> G_NEW/1

== system COSTEP_Auto/Random number generator/Stream Measurements SMEAS Gas analysis/If Action Subsystem3/Subsystem/Stream 13/Subsystem/TESUB6 XMNSEA ==
  G : Inport
  Process Noise I=1-12 G New : mylib/Process Noise I=1-12 G New  SystemSampleTime=-1  VariantActivationTime=update diagram  AllowFlexibleInterface=on  Latency=0  AutoFrameSizeCalculation=off
  XNSEA : Constant  Value=0.25
  XMNSEA : Outport  VectorParamsAs1DForOutWhenUnconnected=off
  G_NEW : Outport  Port=2  VectorParamsAs1DForOutWhenUnconnected=off
  wires:
  XNSEA/1 -> Process Noise I=1-12 G New/1
  Process Noise I=1-12 G New/1 -> XMNSEA/1
  G/1 -> Process Noise I=1-12 G New/2
  Process Noise I=1-12 G New/2 -> G_NEW/1

== system COSTEP_Auto/Random number generator/Stream Measurements SMEAS Gas analysis/If Action Subsystem3/Subsystem/Stream 13/Subsystem/TESUB6 XMNSEB ==
  G : Inport
  Process Noise I=1-12 G New : mylib/Process Noise I=1-12 G New  SystemSampleTime=-1  VariantActivationTime=update diagram  AllowFlexibleInterface=on  Latency=0  AutoFrameSizeCalculation=off
  XNSEB : Constant  Value=0.1
  XMNSEB : Outport  VectorParamsAs1DForOutWhenUnconnected=off
  G_NEW : Outport  Port=2  VectorParamsAs1DForOutWhenUnconnected=off
  wires:
  XNSEB/1 -> Process Noise I=1-12 G New/1
  Process Noise I=1-12 G New/1 -> XMNSEB/1
  G/1 -> Process Noise I=1-12 G New/2
  Process Noise I=1-12 G New/2 -> G_NEW/1

== system COSTEP_Auto/Random number generator/Stream Measurements SMEAS Gas analysis/If Action Subsystem3/Subsystem/Stream 13/Subsystem/TESUB6 XMNSEC ==
  G : Inport
  Process Noise I=1-12 G New : mylib/Process Noise I=1-12 G New  SystemSampleTime=-1  VariantActivationTime=update diagram  AllowFlexibleInterface=on  Latency=0  AutoFrameSizeCalculation=off
  XNSEC : Constant  Value=0.25
  XMNSEC : Outport  VectorParamsAs1DForOutWhenUnconnected=off
  G_NEW : Outport  Port=2  VectorParamsAs1DForOutWhenUnconnected=off
  wires:
  XNSEC/1 -> Process Noise I=1-12 G New/1
  Process Noise I=1-12 G New/1 -> XMNSEC/1
  G/1 -> Process Noise I=1-12 G New/2
  Process Noise I=1-12 G New/2 -> G_NEW/1

== system COSTEP_Auto/Random number generator/Stream Measurements SMEAS Gas analysis/If Action Subsystem3/Subsystem/Stream 13/Subsystem/TESUB6 XMNSED ==
  G : Inport
  Process Noise I=1-12 G New : mylib/Process Noise I=1-12 G New  SystemSampleTime=-1  VariantActivationTime=update diagram  AllowFlexibleInterface=on  Latency=0  AutoFrameSizeCalculation=off
  XNSED : Constant  Value=0.1
  XMNSED : Outport  VectorParamsAs1DForOutWhenUnconnected=off
  G_NEW : Outport  Port=2  VectorParamsAs1DForOutWhenUnconnected=off
  wires:
  XNSED/1 -> Process Noise I=1-12 G New/1
  Process Noise I=1-12 G New/1 -> XMNSED/1
  G/1 -> Process Noise I=1-12 G New/2
  Process Noise I=1-12 G New/2 -> G_NEW/1

== system COSTEP_Auto/Random number generator/Stream Measurements SMEAS Gas analysis/If Action Subsystem3/Subsystem/Stream 13/Subsystem/TESUB6 XMNSEE ==
  G : Inport
  Process Noise I=1-12 G New : mylib/Process Noise I=1-12 G New  SystemSampleTime=-1  VariantActivationTime=update diagram  AllowFlexibleInterface=on  Latency=0  AutoFrameSizeCalculation=off
  XNSEE : Constant  Value=0.25
  XMNSEE : Outport  VectorParamsAs1DForOutWhenUnconnected=off
  G_NEW : Outport  Port=2  VectorParamsAs1DForOutWhenUnconnected=off
  wires:
  XNSEE/1 -> Process Noise I=1-12 G New/1
  Process Noise I=1-12 G New/1 -> XMNSEE/1
  G/1 -> Process Noise I=1-12 G New/2
  Process Noise I=1-12 G New/2 -> G_NEW/1

== system COSTEP_Auto/Random number generator/Stream Measurements SMEAS Gas analysis/If Action Subsystem3/Subsystem/Stream 13/Subsystem/TESUB6 XMNSEF ==
  G : Inport
  Process Noise I=1-12 G New : mylib/Process Noise I=1-12 G New  SystemSampleTime=-1  VariantActivationTime=update diagram  AllowFlexibleInterface=on  Latency=0  AutoFrameSizeCalculation=off
  XNSEF : Constant  Value=0.025
  XMNSEF : Outport  VectorParamsAs1DForOutWhenUnconnected=off
  G_NEW : Outport  Port=2  VectorParamsAs1DForOutWhenUnconnected=off
  wires:
  XNSEF/1 -> Process Noise I=1-12 G New/1
  Process Noise I=1-12 G New/1 -> XMNSEF/1
  G/1 -> Process Noise I=1-12 G New/2
  Process Noise I=1-12 G New/2 -> G_NEW/1

== system COSTEP_Auto/Random number generator/Stream Measurements SMEAS Gas analysis/If Action Subsystem3/Subsystem/Stream 13/Subsystem/TESUB6 XMNSEG ==
  G : Inport
  Process Noise I=1-12 G New : mylib/Process Noise I=1-12 G New  SystemSampleTime=-1  VariantActivationTime=update diagram  AllowFlexibleInterface=on  Latency=0  AutoFrameSizeCalculation=off
  XNSEG : Constant  Value=0.05
  XMNSEG : Outport  VectorParamsAs1DForOutWhenUnconnected=off
  G_NEW : Outport  Port=2  VectorParamsAs1DForOutWhenUnconnected=off
  wires:
  XNSEG/1 -> Process Noise I=1-12 G New/1
  Process Noise I=1-12 G New/1 -> XMNSEG/1
  G/1 -> Process Noise I=1-12 G New/2
  Process Noise I=1-12 G New/2 -> G_NEW/1
